simulink model "Exercise3"  (R2018a)
settings: Solver=VariableStepAuto  StartTime=0.0  StopTime=10  RelTol=1e-3
libraries: dspsrcs4 x3
settings Model: Creator=D18124645  LastModifiedBy=D18124645

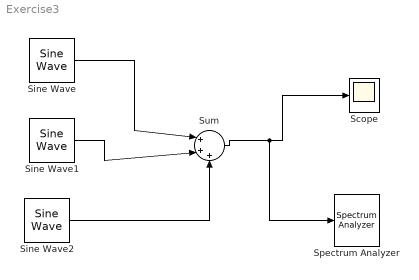
== system Exercise3 ==
  Scope : Scope  NumInputPorts=3
  Sine Wave : dspsrcs4/Sine Wave  Amplitude=1  Frequency=5  Phase=0  SampleMode=Discrete  OutComplex=Real  CompMethod=Trigonometric fcn  TableSize=Speed  SampleTime=1/200  SamplesPerFrame=1  ResetState=Restart at time zero  OutputFrames=off  dataType=double  wordLen=16  udDataType=sfix(16)  fracBitsMode=Best precision  numFracBits=15  OutDataTypeStr=double  LastOutDataTypeStr=double
  Sine Wave1 : dspsrcs4/Sine Wave  Amplitude=1/3  Frequency=5*3  Phase=0  SampleMode=Discrete  OutComplex=Real  CompMethod=Trigonometric fcn  TableSize=Speed  SampleTime=1/200  SamplesPerFrame=1  ResetState=Restart at time zero  OutputFrames=off  dataType=double  wordLen=16  udDataType=sfix(16)  fracBitsMode=Best precision  numFracBits=15  OutDataTypeStr=double  LastOutDataTypeStr=double
  Sine Wave2 : dspsrcs4/Sine Wave  Amplitude=1/5  Frequency=5*5  Phase=0  SampleMode=Discrete  OutComplex=Real  CompMethod=Trigonometric fcn  TableSize=Speed  SampleTime=1/200  SamplesPerFrame=1  ResetState=Restart at time zero  OutputFrames=off  dataType=double  wordLen=16  udDataType=sfix(16)  fracBitsMode=Best precision  numFracBits=15  OutDataTypeStr=double  LastOutDataTypeStr=double
  Spectrum Analyzer : SpectrumAnalyzer
  Sum : Sum  Inputs=|+++
  wires:
  Sine Wave/1 -> Sum/1
  Sine Wave1/1 -> Sum/2
  Sine Wave2/1 -> Sum/3
  Sum/1 -> Spectrum Analyzer/1, Scope/2
